simulink model "zeroSetpointLQR"  (R2019b)
settings: Solver=VariableStepAuto  StartTime=0.0  StopTime=10.0  RelTol=1e-3
values from neighbouring files (symbols this model uses):
  A = [-0.01357  -32.2  -46.3  0 ... (first row only)    [KalmanFilter.m]    (also in LQRwithObserver.m = [-0.01357 -32.2 -46.3 0; part1a.m = [-0.01357 -32.2 -46.3 0)
  B = [-0.433; 0.1394; -0.1394; -0.1577]    [KalmanFilter.m]    (also in LQRwithObserver.m = [-0.433;0.1394;-0.1394;-0.1577]; part1a.m = [-0.433;0.1394;-0.1394;-0.1577])
  C = [0 0 0 1 ... (first row only)    [KalmanFilter.m]    (also in LQRwithObserver.m = eye(n); part1a.m = eye(n))
  x0 = [1 1 1 1]'    [KalmanFilter.m]    (also in LQRwithObserver.m = [1;1;1;1]; part1a.m = [1;1;1;1])
undefined symbols (not defined in the file or in its folder): Fopt
settings Model: Creator=Joseph Shenouda  LastModifiedBy=Joseph Shenouda

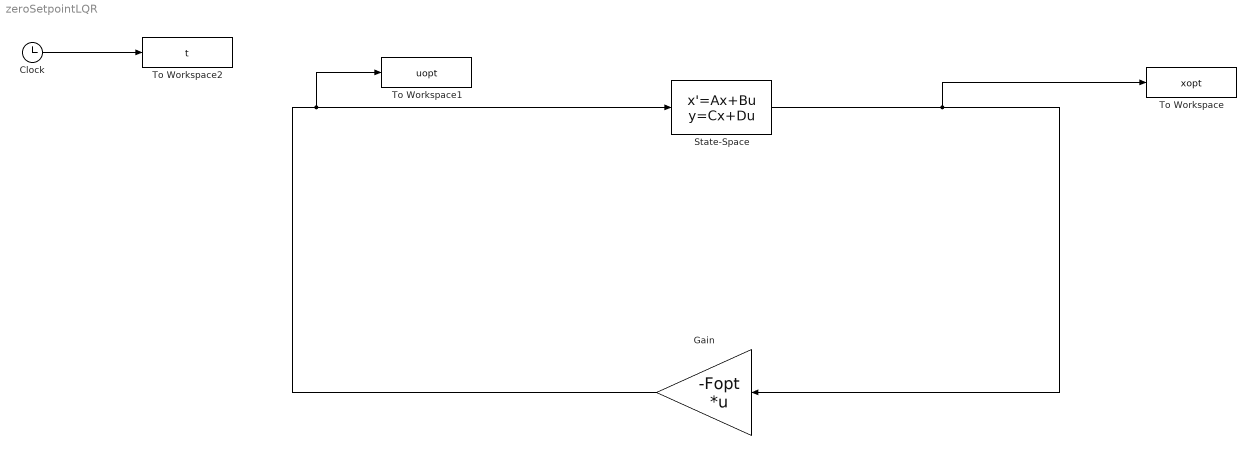
== system zeroSetpointLQR ==
  Clock : Clock
  Gain : Gain  Gain=-Fopt  Multiplication=Matrix(K*u)
  State-Space : StateSpace  A=A  B=B  C=C  D=zeros(4,1)  InitialCondition=x0
  To Workspace : ToWorkspace  VariableName=xopt  SampleTime=-1
  To Workspace1 : ToWorkspace  VariableName=uopt  SampleTime=-1
  To Workspace2 : ToWorkspace  VariableName=t  SampleTime=-1
  wires:
  State-Space/1 -> To Workspace/1, Gain/1
  Gain/1 -> To Workspace1/1, State-Space/1
  Clock/1 -> To Workspace2/1
